simulink model "gm_sampleModel1924_5_sub"  (R2023a)
settings: Solver=VariableStepAuto  StartTime=0.0  StopTime=10.0  RelTol=1e-3
libraries: simulink x2, hdlsllib x1
settings Model: Creator=user1  LastModifiedBy=user1
settings OptimizationCC: BlockReduction=off  ConditionallyExecuteInputs=off
settings DebuggingCC: InheritedTsInSrcMsg=none

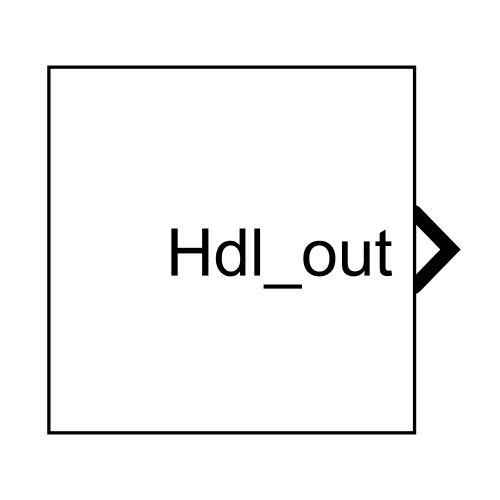
[thumbnail: Simulink's stored preview of the top-level diagram]
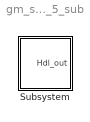
== system gm_sampleModel1924_5_sub ==
  Subsystem : Subsystem

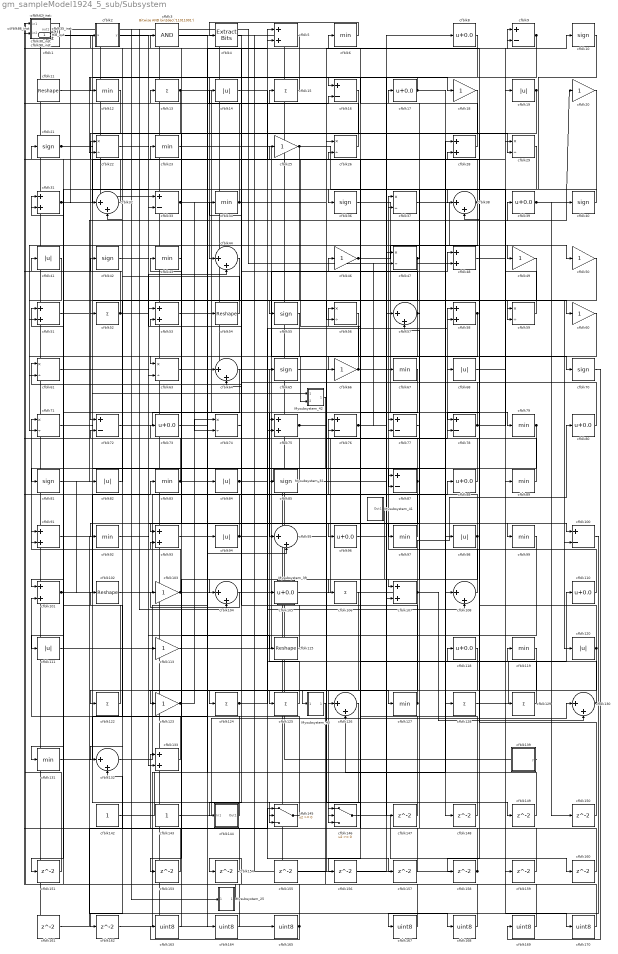
== system gm_sampleModel1924_5_sub/Subsystem ==
  Mysubsystem_25 : Subsystem
  Mysubsystem_32 : Subsystem
  Mysubsystem_39 : Subsystem
  Mysubsystem_40 : Subsystem
  Mysubsystem_41 : Subsystem
  Mysubsystem_42 : Subsystem
  cfblk1 : hdlsllib/Logic and Bit Operations/Interval Test  IntervalClosedRight=on  uplimit=0.5  IntervalClosedLeft=on  lowlimit=-0.5  OutDataTypeStr=uint8
  cfblk{10,21,36,40,42,55,65,70,81,85} (10 alike) : Signum
  cfblk{9,16,33,72,76..78,87,100} (9 alike) : Sum  Inputs=+-  OutDataTypeStr=uint8
  cfblk{5,28,31,48,51,53,58,75,91,93,101,107,133} (13 alike) : Sum  OutDataTypeStr=uint8
  cfblk{11,54,102,115} (4 alike) : Reshape
  cfblk{18,20,25,46,49..50,60,66,103,113,123} (11 alike) : Gain  OutDataTypeStr=uint8
  cfblk{32,38,44,57,64,95,104,108,126,130,132} (11 alike) : Sum  Inputs=|++  OutDataTypeStr=uint8
  cfblk{8,17,39,73,80,88,96,105,110,118} (10 alike) : Bias  Bias=0.0  SaturateOnIntegerOverflow=off
  cfblk{13,15,52,106,122,124..125,128..129} (9 alike) : Sum  Inputs=+  OutDataTypeStr=uint8
  cfblk109_inst : Subsystem
  cfblk{14,19,41,68,82,84,94,98,111,120} (10 alike) : Abs  OutDataTypeStr=uint8  SaturateOnIntegerOverflow=off
  cfblk{6,12,23,34,43,67,79,83,89,92,97,99,119,127,131} (15 alike) : MinMax  OutDataTypeStr=uint8
  cfblk121_inst : Subsystem
  cfblk139 : Subsystem  mask(Counter Free-Running){NumBits=double(16), tsamp=double(-1)}
      mask prompts: NumBits "Simulink:masks:NumberOfBits_MP"; tsamp "Simulink:masks:SampleTime_MP"
      mask help: Simulink:masks:CounterFreeRunning_MD
  cfblk142 : Constant  OutDataTypeStr=uint8  SampleTime=-1
  cfblk143 : Constant  OutDataTypeStr=uint8  SampleTime=-1
  cfblk144 : Subsystem
  cfblk145 : Switch  OutDataTypeStr=uint8  SaturateOnIntegerOverflow=off  InputSameDT=off
  cfblk146 : Switch  OutDataTypeStr=uint8  SaturateOnIntegerOverflow=off  InputSameDT=off
  cfblk{147..151,153..162} (15 alike) : Delay  SampleTime=1
  cfblk{163..165,167..170} (7 alike) : DataTypeConversion  OutDataTypeStr=uint8  SaturateOnIntegerOverflow=off  RndMeth=Floor
  cfblk2 : Subsystem  mask(Compare To Constant){relop=<=, const=double(3), OutDataTypeStr=uint8, ZeroCross=on}
      mask prompts: relop "Simulink:masks:Operator_MP"; const "Simulink:masks:ConstantValue_MP"; OutDataTypeStr "Simulink:masks:OutputDataType_MP"; ZeroCross "Simulink:masks:EnableZerocrossingDetection_MP"
      mask help: Simulink:masks:CompareToConstant_MD
      mask init:
      | OutDataTypeStr = 'uint8';
      | ZeroCross = 'on';
      | blkName = 'sampleModel1924_5_sub/Subsystem/cfblk2';
      | const = double(3);
      | const_str = '3.0';
      | const_val = double(3);
      | relop = '<=';
      | setValue = 'fixdt(0, 8)';
      | str = '<= 3';
      mask TypeOptions relop: == | ~= | < | <= | >= | >
      mask TypeOptions OutDataTypeStr: Simulink:masks:uint8 | Simulink:masks:boolean
      mask Callback ZeroCross: sl('zeroCrossEnable', gcbh);
      mask Display: disp(str)
  cfblk{22,26,29,37,47,56,59,61,63,71,74} (11 alike) : Product  Inputs=*/  OutDataTypeStr=uint8  RndMeth=Zero  SaturateOnIntegerOverflow=on
  cfblk27_inst : Subsystem
  cfblk3 : simulink/Logic and Bit Operations/Bitwise Operator  logicop=AND  UseBitMask=on  BitMask=bin2dec('11011001')  BitMaskRealWorld=Stored Integer
      settings: LibrarySourceBlock=|
      | hdlsllib/Logic and Bit
      | Operations/Bitwise
      | Operator
  cfblk30_inst : Subsystem
  cfblk35_inst : Subsystem
  cfblk4 : simulink/Logic and Bit Operations/Extract Bits  bitsToExtract=Upper half  numBits=8  bitIdxRange=[0 7]  outScalingMode=Preserve fixed-point scaling
      settings: LibrarySourceBlock=|
      | hdlsllib/Logic and Bit
      | Operations/Extract Bits
  cfblk62_inst : Subsystem
  cfblk86_inst : Subsystem
  cfblk90_inst : Subsystem
  Hdl_out : Outport  OutDataTypeStr=uint8  SampleTime=1
  wires:
  Mysubsystem_25/1(Out1) -> cfblk121_inst/1(in1)
  Mysubsystem_32/1(Out1) -> cfblk155/1
  Mysubsystem_39/1(Out1) -> cfblk130/2
  Mysubsystem_40/1(Out1) -> cfblk154/1
  Mysubsystem_41/1(Out1) -> cfblk104/1
  Mysubsystem_42/1(Out1) -> Mysubsystem_32/1(In1)
  cfblk1/1 -> cfblk145/3, cfblk29/2, cfblk18/1, Mysubsystem_42/1(In1)
  cfblk10/1 -> cfblk36/1
  cfblk100/1 -> cfblk167/1
  cfblk101/1 -> cfblk82/1, cfblk83/1
  cfblk102/1 -> cfblk76/1
  cfblk103/1 -> cfblk88/1, cfblk71/1, cfblk15/1
  cfblk104/1 -> cfblk103/1
  cfblk105/1 -> cfblk58/1
  cfblk106/1 -> cfblk122/1
  cfblk107/1 -> cfblk80/1, cfblk146/3
  cfblk108/1 -> cfblk37/1
  cfblk109_inst/1(out1) -> cfblk33/1
  cfblk11/1 -> cfblk33/2
  cfblk110/1 -> cfblk77/1
  cfblk111/1 -> cfblk16/2
  cfblk113/1 -> cfblk48/1
  cfblk115/1 -> cfblk53/2
  cfblk118/1 -> cfblk125/1
  cfblk119/1 -> cfblk162/1
  cfblk12/1 -> cfblk72/1
  cfblk120/1 -> cfblk62_inst/1(in1), cfblk156/1
  cfblk121_inst/1(out1) -> cfblk165/1
  cfblk122/1 -> cfblk51/1
  cfblk123/1 -> cfblk93/2, cfblk74/1
  cfblk124/1 -> cfblk58/2, cfblk119/1
  cfblk125/1 -> cfblk65/1
  cfblk126/1 -> cfblk145/2
  cfblk127/1 -> cfblk53/1, cfblk61/1
  cfblk128/1 -> cfblk110/1
  cfblk129/1 -> cfblk118/1
  cfblk13/1 -> cfblk95/1, cfblk52/1
  cfblk130/1 -> cfblk68/1, cfblk46/1
  cfblk131/1 -> cfblk84/1
  cfblk132/1 -> cfblk54/1
  cfblk133/1 -> cfblk102/1
  cfblk139/1(y) -> cfblk1/1
  cfblk14/1 -> cfblk157/1
  cfblk142/1 -> cfblk28/1
  cfblk143/1 -> cfblk130/1
  cfblk144/1(Out1) -> cfblk13/1
  cfblk145/1 -> cfblk101/2
  cfblk146/1 -> cfblk160/1
  cfblk147/1 -> cfblk75/1
  cfblk148/1 -> cfblk22/1
  cfblk149/1 -> cfblk126/2
  cfblk15/1 -> cfblk12/1
  cfblk150/1 -> cfblk38/2
  cfblk151/1 -> cfblk109_inst/2(in2)
  cfblk153/1 -> cfblk132/2
  cfblk154/1 -> cfblk133/1
  cfblk155/1 -> cfblk9/1
  cfblk156/1 -> cfblk78/2
  cfblk157/1 -> cfblk76/2
  cfblk158/1 -> cfblk57/2, Hdl_out/1
  cfblk159/1 -> cfblk86_inst/2(in2)
  cfblk16/1 -> cfblk124/1
  cfblk160/1 -> cfblk56/1
  cfblk161/1 -> cfblk145/1
  cfblk162/1 -> cfblk64/1
  cfblk163/1 -> cfblk3/1
  cfblk164/1 -> cfblk23/1
  cfblk165/1 -> cfblk163/1, cfblk43/1
  cfblk167/1 -> cfblk121_inst/2(in2)
  cfblk168/1 -> cfblk90_inst/1(in1)
  cfblk169/1 -> cfblk91/1
  cfblk17/1 -> cfblk16/1, cfblk59/2
  cfblk170/1 -> cfblk91/2
  cfblk18/1 -> cfblk133/2
  cfblk19/1 -> cfblk63/1, cfblk158/1
  cfblk2/1(y) -> cfblk115/1
  cfblk20/1 -> cfblk151/1
  cfblk21/1 -> cfblk100/2, cfblk60/1, cfblk128/1
  cfblk22/1 -> cfblk56/2
  cfblk23/1 -> cfblk98/1
  cfblk25/1 -> cfblk63/2, cfblk147/1, cfblk89/1
  cfblk26/1 -> cfblk62_inst/2(in2)
  cfblk27_inst/1(out1) -> cfblk11/1, cfblk161/1
  cfblk28/1 -> cfblk6/1
  cfblk29/1 -> cfblk87/2
  cfblk3/1 -> cfblk164/1
  cfblk30_inst/1(out1) -> cfblk35_inst/1(in1)
  cfblk31/1 -> cfblk5/2, cfblk19/1, cfblk159/1
  cfblk32/1 -> cfblk109_inst/1(in1)
  cfblk33/1 -> cfblk120/1, cfblk74/2
  cfblk34/1 -> cfblk9/2, cfblk30_inst/2(in2)
  cfblk35_inst/1(out1) -> cfblk48/2
  cfblk36/1 -> cfblk148/1
  cfblk37/1 -> cfblk49/1
  cfblk38/1 -> cfblk30_inst/1(in1), cfblk71/2, cfblk66/1
  cfblk39/1 -> cfblk20/1, cfblk150/1
  cfblk4/1 -> cfblk144/1(In1)
  cfblk40/1 -> cfblk38/1
  cfblk41/1 -> cfblk51/2
  cfblk42/1 -> cfblk126/1
  cfblk43/1 -> cfblk93/1
  cfblk44/1 -> cfblk132/1
  cfblk46/1 -> cfblk59/1, cfblk50/1
  cfblk47/1 -> cfblk55/1, cfblk17/1
  cfblk48/1 -> cfblk170/1
  cfblk49/1 -> cfblk87/1
  cfblk5/1 -> cfblk44/1
  cfblk50/1 -> cfblk101/1
  cfblk51/1 -> cfblk39/1
  cfblk52/1 -> cfblk86_inst/1(in1), cfblk44/2
  cfblk53/1 -> cfblk94/1
  cfblk54/1 -> cfblk32/2
  cfblk55/1 -> cfblk64/2
  cfblk56/1 -> cfblk75/2
  cfblk57/1 -> cfblk27_inst/1(in1), cfblk61/2, cfblk97/1
  cfblk58/1 -> Mysubsystem_42/2(In2), cfblk131/1
  cfblk59/1 -> cfblk29/1
  cfblk6/1 -> cfblk4/1
  cfblk60/1 -> cfblk78/1
  cfblk61/1 -> cfblk99/1
  cfblk62_inst/1(out1) -> cfblk35_inst/2(in2), cfblk105/1, cfblk67/1
  cfblk63/1 -> cfblk5/1
  cfblk64/1 -> cfblk111/1
  cfblk65/1 -> cfblk127/1
  cfblk66/1 -> cfblk70/1, cfblk25/1
  cfblk67/1 -> cfblk106/1
  cfblk68/1 -> cfblk129/1
  cfblk70/1 -> cfblk169/1
  cfblk71/1 -> cfblk108/1
  cfblk72/1 -> cfblk79/1
  cfblk73/1 -> cfblk96/1
  cfblk74/1 -> cfblk14/1
  cfblk75/1 -> cfblk77/2, cfblk40/1
  cfblk76/1 -> cfblk8/1, cfblk47/2, cfblk26/2
  cfblk77/1 -> cfblk107/1
  cfblk78/1 -> cfblk10/1, cfblk34/1
  cfblk79/1 -> cfblk81/1, cfblk146/2
  cfblk8/1 -> cfblk22/2
  cfblk80/1 -> cfblk28/2
  cfblk81/1 -> cfblk37/2
  cfblk82/1 -> cfblk2/1(u)
  cfblk83/1 -> cfblk85/1, cfblk72/2, cfblk41/1, cfblk27_inst/2(in2)
  cfblk84/1 -> cfblk100/1, Mysubsystem_40/1(In1)
  cfblk85/1 -> cfblk73/1, cfblk47/1
  cfblk86_inst/1(out1) -> cfblk32/1, cfblk104/2
  cfblk87/1 -> cfblk31/1, cfblk92/1
  cfblk88/1 -> cfblk26/1
  cfblk89/1 -> cfblk42/1
  cfblk9/1 -> cfblk146/1, cfblk107/2
  cfblk90_inst/1(out1) -> Mysubsystem_25/1(In1)
  cfblk91/1 -> cfblk168/1
  cfblk92/1 -> cfblk113/1
  cfblk93/1 -> cfblk95/2
  cfblk94/1 -> cfblk31/2, cfblk108/2
  cfblk95/1 -> cfblk149/1
  cfblk96/1 -> cfblk57/1
  cfblk97/1 -> cfblk21/1
  cfblk98/1 -> cfblk90_inst/2(in2), cfblk153/1
  cfblk99/1 -> cfblk123/1

== system gm_sampleModel1924_5_sub/Subsystem/Mysubsystem_25 ==
  In1 : Inport  OutDataTypeStr=uint8  PortDimensions=1  SampleTime=1
  cfblk152 : Delay  SampleTime=1
  cfblk166 : DataTypeConversion  OutDataTypeStr=uint8  SaturateOnIntegerOverflow=off  RndMeth=Floor
  Out1 : Outport  SampleTime=1
  wires:
  In1/1 -> cfblk152/1
  cfblk152/1 -> cfblk166/1
  cfblk166/1 -> Out1/1

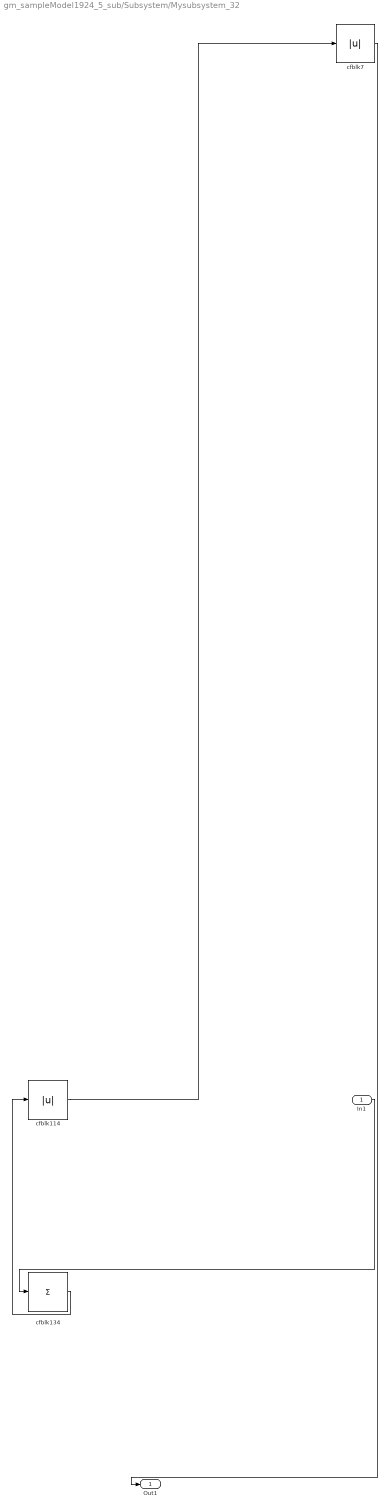
== system gm_sampleModel1924_5_sub/Subsystem/Mysubsystem_32 ==
  In1 : Inport  OutDataTypeStr=uint8  PortDimensions=1  SampleTime=1
  cfblk114 : Abs  SaturateOnIntegerOverflow=off
  cfblk134 : Sum  Inputs=+
  cfblk7 : Abs  SaturateOnIntegerOverflow=off
  Out1 : Outport  SampleTime=1
  wires:
  In1/1 -> cfblk134/1
  cfblk114/1 -> cfblk7/1
  cfblk134/1 -> cfblk114/1
  cfblk7/1 -> Out1/1

== system gm_sampleModel1924_5_sub/Subsystem/Mysubsystem_39 ==
  cfblk141 : Subsystem  mask(Counter Limited){uplimit=double(7), tsamp=double(-1)}
      mask prompts: uplimit "Simulink:masks:UpperLimit_MP"; tsamp "Simulink:masks:SampleTime_MP"
      mask help: Simulink:masks:CounterLimited_MD
      mask init:
      | nbits = double(8);
      | tsamp = double(-1);
      | uplimit = double(7);
  cfblk69 : MinMax
  Out1 : Outport  SampleTime=1
  wires:
  cfblk141/1(y) -> cfblk69/1
  cfblk69/1 -> Out1/1

== system gm_sampleModel1924_5_sub/Subsystem/Mysubsystem_40 ==
  In1 : Inport  OutDataTypeStr=uint8  PortDimensions=1  SampleTime=1
  cfblk116 : Abs  SaturateOnIntegerOverflow=off
  cfblk135 : Signum
  Out1 : Outport  SampleTime=1
  wires:
  In1/1 -> cfblk116/1
  cfblk116/1 -> cfblk135/1
  cfblk135/1 -> Out1/1

== system gm_sampleModel1924_5_sub/Subsystem/Mysubsystem_41 ==
  cfblk138 : Subsystem  mask(Counter Free-Running){NumBits=double(16), tsamp=double(-1)}
      mask prompts: NumBits "Simulink:masks:NumberOfBits_MP"; tsamp "Simulink:masks:SampleTime_MP"
      mask help: Simulink:masks:CounterFreeRunning_MD
  cfblk45 : Signum
  Out1 : Outport  SampleTime=1
  wires:
  cfblk138/1(y) -> cfblk45/1
  cfblk45/1 -> Out1/1

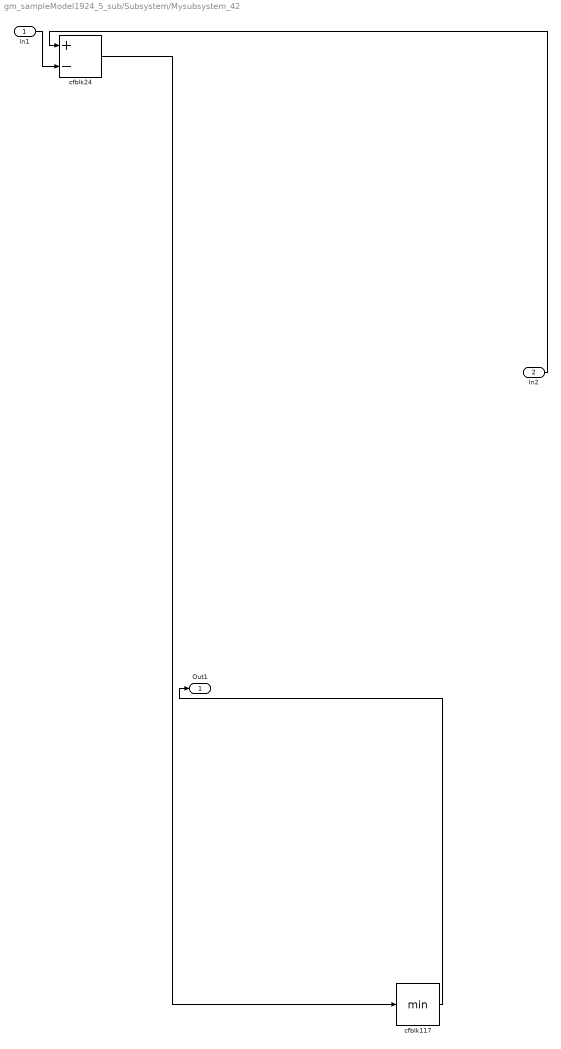
== system gm_sampleModel1924_5_sub/Subsystem/Mysubsystem_42 ==
  In1 : Inport  OutDataTypeStr=uint8  PortDimensions=1  SampleTime=1
  In2 : Inport  Port=2  OutDataTypeStr=uint8  PortDimensions=1  SampleTime=1
  cfblk117 : MinMax
  cfblk24 : Sum  Inputs=+-
  Out1 : Outport  SampleTime=1
  wires:
  In1/1 -> cfblk24/2
  In2/1 -> cfblk24/1
  cfblk117/1 -> Out1/1
  cfblk24/1 -> cfblk117/1

== system gm_sampleModel1924_5_sub/Subsystem/cfblk109_inst ==
  in1 : Inport  OutDataTypeStr=uint8  SampleTime=1
  in2 : Inport  Port=2  OutDataTypeStr=uint8  SampleTime=1
  mul_cfblk109_dotp_mulcomp : Product  Inputs=**  OutDataTypeStr=uint8  SampleTime=1
  out1 : Outport  OutDataTypeStr=uint8  SampleTime=1
  wires:
  in1/1 -> mul_cfblk109_dotp_mulcomp/1
  in2/1 -> mul_cfblk109_dotp_mulcomp/2
  mul_cfblk109_dotp_mulcomp/1 -> out1/1

== system gm_sampleModel1924_5_sub/Subsystem/cfblk121_inst ==
  in1 : Inport  OutDataTypeStr=uint8  SampleTime=1
  in2 : Inport  Port=2  OutDataTypeStr=uint8  SampleTime=1
  mul_cfblk121_dotp_mulcomp : Product  Inputs=**  OutDataTypeStr=uint8  SampleTime=1
  out1 : Outport  OutDataTypeStr=uint8  SampleTime=1
  wires:
  in1/1 -> mul_cfblk121_dotp_mulcomp/1
  in2/1 -> mul_cfblk121_dotp_mulcomp/2
  mul_cfblk121_dotp_mulcomp/1 -> out1/1

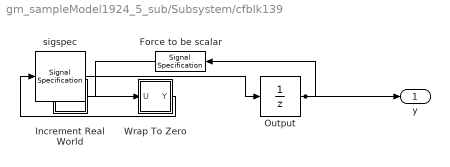
== system gm_sampleModel1924_5_sub/Subsystem/cfblk139 ==
  Force to be scalar : SignalSpecification  DisableCoverage=on  Dimensions=1
  Increment Real World : Subsystem  mask(Real World Value Increment){}
      mask help: Simulink:masks:RealWorldValueIncrement_MD
      mask Display: disp('V++')
  Output : UnitDelay  InitialCondition=0.0  SampleTime=tsamp  HasFrameUpgradeWarning=on
  Wrap To Zero : Subsystem  mask(Wrap To Zero){Threshold=double(65535)}
      mask prompts: Threshold "Simulink:masks:Threshold_MP"
      mask help: Simulink:masks:WrapToZero_MD
  sigspec : SignalSpecification  OutDataTypeStr=uint16  Dimensions=1
  y : Outport  SampleTime=1
  wires:
  Force to be scalar/1 -> Increment Real World/1(u)
  Increment Real World/1(y) -> Wrap To Zero/1(U)
  Output/1 -> Force to be scalar/1, y/1
  Wrap To Zero/1(Y) -> sigspec/1
  sigspec/1 -> Output/1

== system gm_sampleModel1924_5_sub/Subsystem/cfblk144 ==
  In1 : Inport  OutDataTypeStr=fixdt(0, 4, -4)  PortDimensions=1  SampleTime=1
  Out1 : Outport  SampleTime=1
  wires:
  In1/1 -> Out1/1

== system gm_sampleModel1924_5_sub/Subsystem/cfblk2 ==
  u : Inport  OutDataTypeStr=uint8  SampleTime=1
  Compare : RelationalOperator  Operator=<=  OutDataTypeStr=fixdt(0, 8)
  Constant : Constant  DisableCoverage=on  Value=const  OutDataTypeStr=Inherit: Inherit via back propagation  SampleTime=-1
  y : Outport  SampleTime=1
  wires:
  u/1 -> Compare/1
  Compare/1 -> y/1
  Constant/1 -> Compare/2

== system gm_sampleModel1924_5_sub/Subsystem/cfblk27_inst ==
  in1 : Inport  OutDataTypeStr=uint8  SampleTime=1
  in2 : Inport  Port=2  OutDataTypeStr=uint8  SampleTime=1
  mul_cfblk27_dotp_mulcomp : Product  Inputs=**  OutDataTypeStr=uint8  SampleTime=1
  out1 : Outport  OutDataTypeStr=uint8  SampleTime=1
  wires:
  in1/1 -> mul_cfblk27_dotp_mulcomp/1
  in2/1 -> mul_cfblk27_dotp_mulcomp/2
  mul_cfblk27_dotp_mulcomp/1 -> out1/1

== system gm_sampleModel1924_5_sub/Subsystem/cfblk30_inst ==
  in1 : Inport  OutDataTypeStr=uint8  SampleTime=1
  in2 : Inport  Port=2  OutDataTypeStr=uint8  SampleTime=1
  mul_cfblk30_dotp_mulcomp : Product  Inputs=**  OutDataTypeStr=uint8  SampleTime=1
  out1 : Outport  OutDataTypeStr=uint8  SampleTime=1
  wires:
  in1/1 -> mul_cfblk30_dotp_mulcomp/1
  in2/1 -> mul_cfblk30_dotp_mulcomp/2
  mul_cfblk30_dotp_mulcomp/1 -> out1/1

== system gm_sampleModel1924_5_sub/Subsystem/cfblk35_inst ==
  in1 : Inport  OutDataTypeStr=uint8  SampleTime=1
  in2 : Inport  Port=2  OutDataTypeStr=uint8  SampleTime=1
  mul_cfblk35_dotp_mulcomp : Product  Inputs=**  OutDataTypeStr=uint8  SampleTime=1
  out1 : Outport  OutDataTypeStr=uint8  SampleTime=1
  wires:
  in1/1 -> mul_cfblk35_dotp_mulcomp/1
  in2/1 -> mul_cfblk35_dotp_mulcomp/2
  mul_cfblk35_dotp_mulcomp/1 -> out1/1

== system gm_sampleModel1924_5_sub/Subsystem/cfblk62_inst ==
  in1 : Inport  OutDataTypeStr=uint8  SampleTime=1
  in2 : Inport  Port=2  OutDataTypeStr=uint8  SampleTime=1
  mul_cfblk62_dotp_mulcomp : Product  Inputs=**  OutDataTypeStr=uint8  SampleTime=1
  out1 : Outport  OutDataTypeStr=uint8  SampleTime=1
  wires:
  in1/1 -> mul_cfblk62_dotp_mulcomp/1
  in2/1 -> mul_cfblk62_dotp_mulcomp/2
  mul_cfblk62_dotp_mulcomp/1 -> out1/1

== system gm_sampleModel1924_5_sub/Subsystem/cfblk86_inst ==
  in1 : Inport  OutDataTypeStr=uint8  SampleTime=1
  in2 : Inport  Port=2  OutDataTypeStr=uint8  SampleTime=1
  mul_cfblk86_dotp_mulcomp : Product  Inputs=**  OutDataTypeStr=uint8  SampleTime=1
  out1 : Outport  OutDataTypeStr=uint8  SampleTime=1
  wires:
  in1/1 -> mul_cfblk86_dotp_mulcomp/1
  in2/1 -> mul_cfblk86_dotp_mulcomp/2
  mul_cfblk86_dotp_mulcomp/1 -> out1/1

== system gm_sampleModel1924_5_sub/Subsystem/cfblk90_inst ==
  in1 : Inport  OutDataTypeStr=uint8  SampleTime=1
  in2 : Inport  Port=2  OutDataTypeStr=uint8  SampleTime=1
  mul_cfblk90_dotp_mulcomp : Product  Inputs=**  OutDataTypeStr=uint8  SampleTime=1
  out1 : Outport  OutDataTypeStr=uint8  SampleTime=1
  wires:
  in1/1 -> mul_cfblk90_dotp_mulcomp/1
  in2/1 -> mul_cfblk90_dotp_mulcomp/2
  mul_cfblk90_dotp_mulcomp/1 -> out1/1

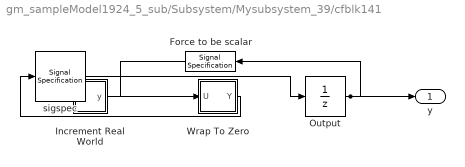
== system gm_sampleModel1924_5_sub/Subsystem/Mysubsystem_39/cfblk141 ==
  Force to be scalar : SignalSpecification  DisableCoverage=on  Dimensions=1
  Increment Real World : Subsystem  mask(Real World Value Increment){}
      mask help: Simulink:masks:RealWorldValueIncrement_MD
      mask Display: disp('V++')
  Output : UnitDelay  InitialCondition=0.0  SampleTime=tsamp  HasFrameUpgradeWarning=on
  Wrap To Zero : Subsystem  mask(Wrap To Zero){Threshold=double(7)}
      mask prompts: Threshold "Simulink:masks:Threshold_MP"
      mask help: Simulink:masks:WrapToZero_MD
  sigspec : SignalSpecification  OutDataTypeStr=uint8  Dimensions=1
  y : Outport  SampleTime=1
  wires:
  Force to be scalar/1 -> Increment Real World/1(u)
  Increment Real World/1(y) -> Wrap To Zero/1(U)
  Output/1 -> Force to be scalar/1, y/1
  Wrap To Zero/1(Y) -> sigspec/1
  sigspec/1 -> Output/1

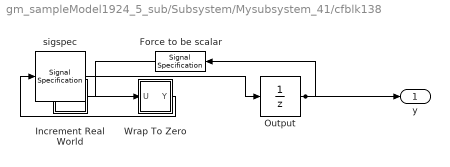
== system gm_sampleModel1924_5_sub/Subsystem/Mysubsystem_41/cfblk138 ==
  Force to be scalar : SignalSpecification  DisableCoverage=on  Dimensions=1
  Increment Real World : Subsystem  mask(Real World Value Increment){}
      mask help: Simulink:masks:RealWorldValueIncrement_MD
      mask Display: disp('V++')
  Output : UnitDelay  InitialCondition=0.0  SampleTime=tsamp  HasFrameUpgradeWarning=on
  Wrap To Zero : Subsystem  mask(Wrap To Zero){Threshold=double(65535)}
      mask prompts: Threshold "Simulink:masks:Threshold_MP"
      mask help: Simulink:masks:WrapToZero_MD
  sigspec : SignalSpecification  OutDataTypeStr=uint16  Dimensions=1
  y : Outport  SampleTime=1
  wires:
  Force to be scalar/1 -> Increment Real World/1(u)
  Increment Real World/1(y) -> Wrap To Zero/1(U)
  Output/1 -> Force to be scalar/1, y/1
  Wrap To Zero/1(Y) -> sigspec/1
  sigspec/1 -> Output/1

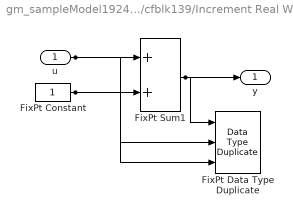
== system gm_sampleModel1924_5_sub/Subsystem/cfblk139/Increment Real World ==
  u : Inport  OutDataTypeStr=uint16  SampleTime=1
  FixPt Constant : Constant  DisableCoverage=on  OutDataTypeStr=Inherit: Inherit via back propagation  SampleTime=-1
  FixPt Data Type Duplicate : DataTypeDuplicate  DisableCoverage=on  NumInputPorts=3
  FixPt Sum1 : Sum  InputSameDT=on  OutDataTypeStr=Inherit: Inherit via back propagation  LockScale=on
  y : Outport  SampleTime=1
  wires:
  u/1 -> FixPt Sum1/1, FixPt Data Type Duplicate/2
  FixPt Constant/1 -> FixPt Sum1/2, FixPt Data Type Duplicate/3
  FixPt Sum1/1 -> FixPt Data Type Duplicate/1, y/1

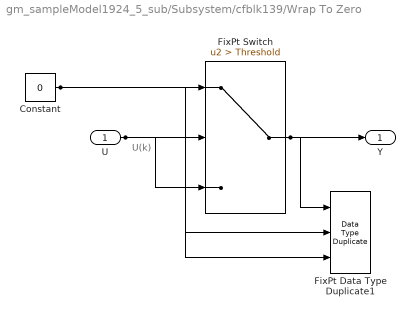
== system gm_sampleModel1924_5_sub/Subsystem/cfblk139/Wrap To Zero ==
  note: U(k)
  U : Inport  OutDataTypeStr=uint16  SampleTime=1
  Constant : Constant  DisableCoverage=on  Value=0  OutDataTypeStr=Inherit: Inherit via back propagation  SampleTime=-1
  FixPt Data Type Duplicate1 : DataTypeDuplicate  DisableCoverage=on  NumInputPorts=3
  FixPt Switch : Switch  Criteria=u2 > Threshold  Threshold=Threshold  OutDataTypeStr=Inherit: Inherit via back propagation  ZeroCross=off  SaturateOnIntegerOverflow=off  InputSameDT=off
  Y : Outport  SampleTime=1
  wires:
  U/1 -> FixPt Switch/3, FixPt Switch/2, FixPt Data Type Duplicate1/2
  Constant/1 -> FixPt Switch/1, FixPt Data Type Duplicate1/3
  FixPt Switch/1 -> FixPt Data Type Duplicate1/1, Y/1

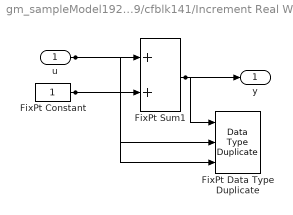
== system gm_sampleModel1924_5_sub/Subsystem/Mysubsystem_39/cfblk141/Increment Real World ==
  u : Inport  OutDataTypeStr=uint8  SampleTime=1
  FixPt Constant : Constant  DisableCoverage=on  OutDataTypeStr=Inherit: Inherit via back propagation  SampleTime=-1
  FixPt Data Type Duplicate : DataTypeDuplicate  DisableCoverage=on  NumInputPorts=3
  FixPt Sum1 : Sum  InputSameDT=on  OutDataTypeStr=Inherit: Inherit via back propagation  LockScale=on
  y : Outport  SampleTime=1
  wires:
  u/1 -> FixPt Sum1/1, FixPt Data Type Duplicate/2
  FixPt Constant/1 -> FixPt Sum1/2, FixPt Data Type Duplicate/3
  FixPt Sum1/1 -> FixPt Data Type Duplicate/1, y/1

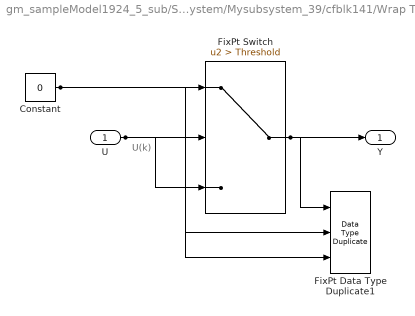
== system gm_sampleModel1924_5_sub/Subsystem/Mysubsystem_39/cfblk141/Wrap To Zero ==
  note: U(k)
  U : Inport  OutDataTypeStr=uint8  SampleTime=1
  Constant : Constant  DisableCoverage=on  Value=0  OutDataTypeStr=Inherit: Inherit via back propagation  SampleTime=-1
  FixPt Data Type Duplicate1 : DataTypeDuplicate  DisableCoverage=on  NumInputPorts=3
  FixPt Switch : Switch  Criteria=u2 > Threshold  Threshold=Threshold  OutDataTypeStr=Inherit: Inherit via back propagation  ZeroCross=off  SaturateOnIntegerOverflow=off  InputSameDT=off
  Y : Outport  SampleTime=1
  wires:
  U/1 -> FixPt Switch/3, FixPt Switch/2, FixPt Data Type Duplicate1/2
  Constant/1 -> FixPt Switch/1, FixPt Data Type Duplicate1/3
  FixPt Switch/1 -> FixPt Data Type Duplicate1/1, Y/1

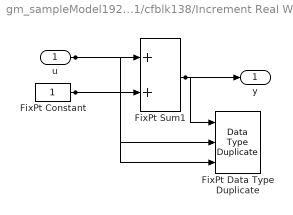
== system gm_sampleModel1924_5_sub/Subsystem/Mysubsystem_41/cfblk138/Increment Real World ==
  u : Inport  OutDataTypeStr=uint16  SampleTime=1
  FixPt Constant : Constant  DisableCoverage=on  OutDataTypeStr=Inherit: Inherit via back propagation  SampleTime=-1
  FixPt Data Type Duplicate : DataTypeDuplicate  DisableCoverage=on  NumInputPorts=3
  FixPt Sum1 : Sum  InputSameDT=on  OutDataTypeStr=Inherit: Inherit via back propagation  LockScale=on
  y : Outport  SampleTime=1
  wires:
  u/1 -> FixPt Sum1/1, FixPt Data Type Duplicate/2
  FixPt Constant/1 -> FixPt Sum1/2, FixPt Data Type Duplicate/3
  FixPt Sum1/1 -> FixPt Data Type Duplicate/1, y/1

== system gm_sampleModel1924_5_sub/Subsystem/Mysubsystem_41/cfblk138/Wrap To Zero ==
  note: U(k)
  U : Inport  OutDataTypeStr=uint16  SampleTime=1
  Constant : Constant  DisableCoverage=on  Value=0  OutDataTypeStr=Inherit: Inherit via back propagation  SampleTime=-1
  FixPt Data Type Duplicate1 : DataTypeDuplicate  DisableCoverage=on  NumInputPorts=3
  FixPt Switch : Switch  Criteria=u2 > Threshold  Threshold=Threshold  OutDataTypeStr=Inherit: Inherit via back propagation  ZeroCross=off  SaturateOnIntegerOverflow=off  InputSameDT=off
  Y : Outport  SampleTime=1
  wires:
  U/1 -> FixPt Switch/3, FixPt Switch/2, FixPt Data Type Duplicate1/2
  Constant/1 -> FixPt Switch/1, FixPt Data Type Duplicate1/3
  FixPt Switch/1 -> FixPt Data Type Duplicate1/1, Y/1
